simulink model "TESTPIDSIMULIN"  (R2024b)
settings: Solver=VariableStepAuto  StartTime=0.0  StopTime=5  RelTol=1e-3
settings Model: Creator=miao
settings OptimizationCC: ReuseModelBlockBuffer=off
settings RTWCC: GPUComputeCapability=3.5

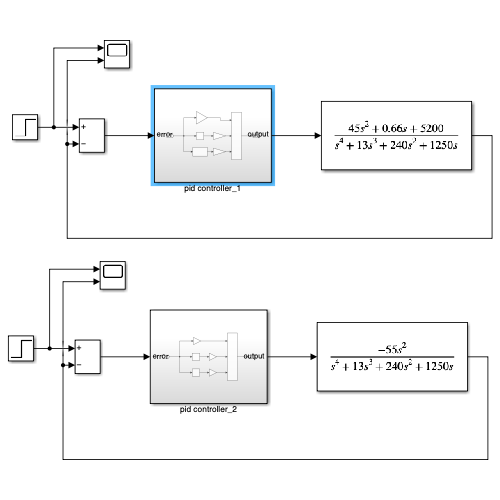
[thumbnail: Simulink's stored preview of the top-level diagram]
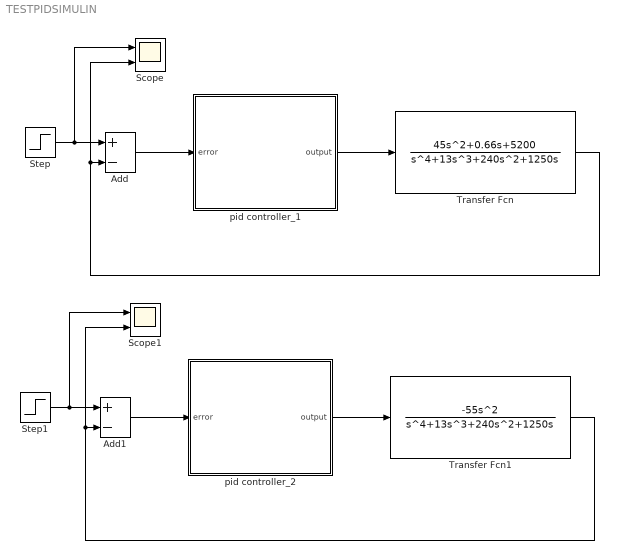
== system TESTPIDSIMULIN ==
  Add : Sum  Inputs=+-
  Add1 : Sum  Inputs=+-
  Scope : Scope  NumInputPorts=2
  Scope1 : Scope  NumInputPorts=2
  Step : Step  SampleTime=0
  Step1 : Step  SampleTime=0
  Transfer Fcn : TransferFcn  Numerator=[45 0.66 5200]  Denominator=[1 13 240 1250 0]
  Transfer Fcn1 : TransferFcn  Numerator=[-55 0 0]  Denominator=[1 13 240 1250 0]
  pid controller_1 : Subsystem
  pid controller_2 : Subsystem
  wires:
  pid controller_1/1(output) -> Transfer Fcn/1
  Step/1 -> Scope/1, Add/1
  Transfer Fcn/1 -> Scope/2, Add/2
  Add/1 -> pid controller_1/1(error)
  Add1/1 -> pid controller_2/1(error)
  Transfer Fcn1/1 -> Add1/2, Scope1/2
  Step1/1 -> Add1/1, Scope1/1
  pid controller_2/1(output) -> Transfer Fcn1/1

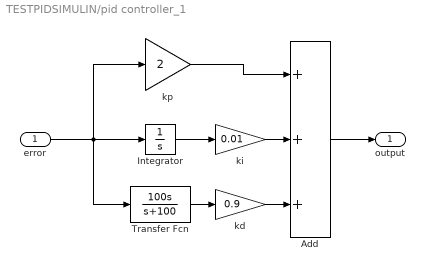
== system TESTPIDSIMULIN/pid controller_1 ==
  error : Inport
  Add : Sum  Inputs=+++
  Integrator : Integrator
  Transfer Fcn : TransferFcn  Numerator=[100 0]  Denominator=[1 100]
  kd : Gain  Gain=0.9
  ki : Gain  Gain=0.01
  kp : Gain  Gain=2
  output : Outport
  wires:
  Integrator/1 -> ki/1
  Transfer Fcn/1 -> kd/1
  kp/1 -> Add/1
  ki/1 -> Add/2
  kd/1 -> Add/3
  Add/1 -> output/1
  error/1 -> Transfer Fcn/1, Integrator/1, kp/1

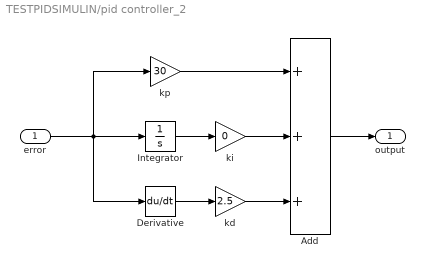
== system TESTPIDSIMULIN/pid controller_2 ==
  error : Inport
  Add : Sum  Inputs=+++
  Derivative : Derivative
  Integrator : Integrator
  kd : Gain  Gain=2.5
  ki : Gain  Gain=0
  kp : Gain  Gain=30
  output : Outport
  wires:
  error/1 -> kp/1, Integrator/1, Derivative/1
  Add/1 -> output/1
  kd/1 -> Add/3
  ki/1 -> Add/2
  kp/1 -> Add/1
  Derivative/1 -> kd/1
  Integrator/1 -> ki/1
